simulink model "Van0"  (R2024b)
settings: Solver=ode3  StartTime=0.0  StopTime=10  FixedStep=0.001  RelTol=1e-3
Description:
  | 原始版本
settings Model: PacingRate=1000  Creator=繁星  LastModifiedBy=14422
settings SolverCC: ShapePreserveControl=EnableAll  ZeroCrossAlgorithm=Adaptive
settings DataIOCC: ReturnWorkspaceOutputs=off
settings OptimizationCC: ReuseModelBlockBuffer=off
settings ModelReferenceCC: EnableRefExpFcnMdlSchedulingChecks=on
settings RTWCC: GPUComputeCapability=3.5

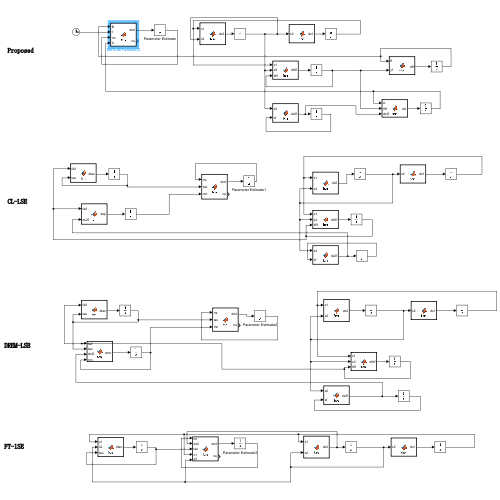
[thumbnail: Simulink's stored preview of the top-level diagram]
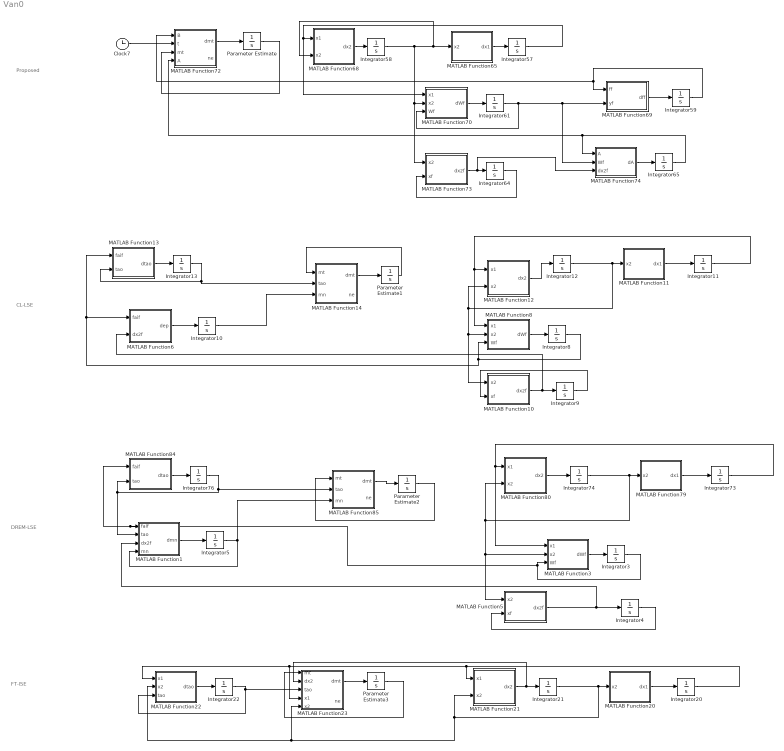
== system Van0 ==
  note: Proposed
  note: CL-LSE
  note: DREM-LSE
  note: FT-lSE
  Clock7 : Clock
  Integrator10 : Integrator  InitialCondition=[0;0;0]
  Integrator{11,20,57,73} (4 alike) : Integrator  InitialCondition=1
  Integrator{3..4,8..9,12,21,58,61,64..65,74} (11 alike) : Integrator
  Integrator13 : Integrator  InitialCondition=1000*eye(3)
  Integrator22 : Integrator  InitialCondition=1000*eye(3)
  Integrator5 : Integrator  InitialCondition=[0;0;0]
  Integrator59 : Integrator  InitialCondition=[1 0 0;0 1 0;0 0 1]*1e-7
  Integrator76 : Integrator  InitialCondition=1000*eye(3)
  MATLAB Function1 : MATLAB Function  TreatAsAtomicUnit=on
  MATLAB Function10 : MATLAB Function  TreatAsAtomicUnit=on
  MATLAB Function11 : MATLAB Function  TreatAsAtomicUnit=on
  MATLAB Function12 : MATLAB Function  TreatAsAtomicUnit=on
  MATLAB Function13 : MATLAB Function  TreatAsAtomicUnit=on
  MATLAB Function14 : MATLAB Function  TreatAsAtomicUnit=on
  MATLAB Function20 : MATLAB Function  TreatAsAtomicUnit=on
  MATLAB Function21 : MATLAB Function  TreatAsAtomicUnit=on
  MATLAB Function22 : MATLAB Function  TreatAsAtomicUnit=on
  MATLAB Function23 : MATLAB Function  TreatAsAtomicUnit=on
  MATLAB Function3 : MATLAB Function  TreatAsAtomicUnit=on
  MATLAB Function5 : MATLAB Function  TreatAsAtomicUnit=on
  MATLAB Function6 : MATLAB Function  TreatAsAtomicUnit=on
  MATLAB Function65 : MATLAB Function  TreatAsAtomicUnit=on
  MATLAB Function68 : MATLAB Function  TreatAsAtomicUnit=on
  MATLAB Function69 : MATLAB Function  TreatAsAtomicUnit=on
  MATLAB Function70 : MATLAB Function  TreatAsAtomicUnit=on
  MATLAB Function72 : MATLAB Function  TreatAsAtomicUnit=on
  MATLAB Function73 : MATLAB Function  TreatAsAtomicUnit=on
  MATLAB Function74 : MATLAB Function  TreatAsAtomicUnit=on
  MATLAB Function79 : MATLAB Function  TreatAsAtomicUnit=on
  MATLAB Function8 : MATLAB Function  TreatAsAtomicUnit=on
  MATLAB Function80 : MATLAB Function  TreatAsAtomicUnit=on
  MATLAB Function84 : MATLAB Function  TreatAsAtomicUnit=on
  MATLAB Function85 : MATLAB Function  TreatAsAtomicUnit=on
  Parameter Estimate : Integrator
  Parameter Estimate1 : Integrator  InitialCondition=[0.5;-1;1]*0
  Parameter Estimate2 : Integrator  InitialCondition=[0.5;-1;1]*0
  Parameter Estimate3 : Integrator  InitialCondition=[0.5;-1;1]*0
  wires:
  MATLAB Function73/1(dx2f) -> MATLAB Function74/3(dx2f), Integrator64/1
  MATLAB Function80/1(dx2) -> Integrator74/1
  MATLAB Function79/1(dx1) -> Integrator73/1
  MATLAB Function84/1(dtao) -> Integrator76/1
  Parameter Estimate2/1 -> MATLAB Function85/1(mt)
  Parameter Estimate/1 -> MATLAB Function72/3(mt)
  Integrator76/1 -> MATLAB Function1/2(tao), MATLAB Function84/2(tao), MATLAB Function85/2(tao)
  MATLAB Function85/1(dmt) -> Parameter Estimate2/1
  MATLAB Function69/1(dff) -> Integrator59/1
  Integrator59/1 -> MATLAB Function72/1(B), MATLAB Function69/1(ff)
  MATLAB Function68/1(dx2) -> Integrator58/1
  MATLAB Function70/1(dWf) -> Integrator61/1
  Integrator61/1 -> MATLAB Function70/3(Wf), MATLAB Function74/2(Wf), MATLAB Function69/2(yf)
  MATLAB Function74/1(dA) -> Integrator65/1
  Integrator65/1 -> MATLAB Function72/4(A), MATLAB Function74/1(A)
  MATLAB Function65/1(dx1) -> Integrator57/1
  Integrator64/1 -> MATLAB Function73/2(xf)
  MATLAB Function72/1(dmt) -> Parameter Estimate/1
  Clock7/1 -> MATLAB Function72/2(t)
  Integrator58/1 -> MATLAB Function68/2(x2), MATLAB Function65/1(x2), MATLAB Function70/2(x2), MATLAB Function73/1(x2)
  MATLAB Function3/1(dWf) -> Integrator3/1
  Integrator4/1 -> MATLAB Function5/2(xf)
  MATLAB Function5/1(dx2f) -> MATLAB Function1/3(dx2f), Integrator4/1
  Integrator3/1 -> MATLAB Function84/1(faif), MATLAB Function1/1(faif), MATLAB Function3/3(Wf)
  MATLAB Function1/1(dmn) -> Integrator5/1
  Integrator5/1 -> MATLAB Function1/4(mn), MATLAB Function85/3(mn)
  Integrator74/1 -> MATLAB Function5/1(x2), MATLAB Function3/2(x2), MATLAB Function80/2(x2), MATLAB Function79/1(x2)
  Integrator9/1 -> MATLAB Function10/2(xf)
  MATLAB Function8/1(dWf) -> Integrator8/1
  MATLAB Function6/1(dep) -> Integrator10/1
  MATLAB Function10/1(dx2f) -> Integrator9/1, MATLAB Function6/2(dx2f)
  Parameter Estimate1/1 -> MATLAB Function14/1(mt)
  MATLAB Function11/1(dx1) -> Integrator11/1
  MATLAB Function14/1(dmt) -> Parameter Estimate1/1
  Integrator12/1 -> MATLAB Function10/1(x2), MATLAB Function8/2(x2), MATLAB Function12/2(x2), MATLAB Function11/1(x2)
  MATLAB Function13/1(dtao) -> Integrator13/1
  Integrator8/1 -> MATLAB Function8/3(Wf), MATLAB Function13/1(faif), MATLAB Function6/1(faif)
  MATLAB Function12/1(dx2) -> Integrator12/1
  Integrator10/1 -> MATLAB Function14/3(mn)
  Integrator22/1 -> MATLAB Function22/3(tao), MATLAB Function23/3(tao)
  Parameter Estimate3/1 -> MATLAB Function23/1(mt)
  MATLAB Function20/1(dx1) -> Integrator20/1
  MATLAB Function23/1(dmt) -> Parameter Estimate3/1
  Integrator21/1 -> MATLAB Function20/1(x2), MATLAB Function23/5(x2), MATLAB Function22/2(x2), MATLAB Function21/2(x2)
  MATLAB Function22/1(dtao) -> Integrator22/1
  MATLAB Function21/1(dx2) -> MATLAB Function23/2(dx2), Integrator21/1
  Integrator13/1 -> MATLAB Function14/2(tao), MATLAB Function13/2(tao)
  Integrator57/1 -> MATLAB Function70/1(x1), MATLAB Function68/1(x1)
  Integrator11/1 -> MATLAB Function8/1(x1), MATLAB Function12/1(x1)
  Integrator73/1 -> MATLAB Function3/1(x1), MATLAB Function80/1(x1)
  Integrator20/1 -> MATLAB Function22/1(x1), MATLAB Function23/4(x1), MATLAB Function21/1(x1)

== matlab function Van0/MATLAB Function8 ==
  data: x1 input; dWf output; x2 input; Wf input
function dWf  = fcn(x1,x2,Wf)

A=[-x1,x2,-x1*x1*x2];
dWf=-0.1*Wf+A;

== matlab function Van0/MATLAB Function20 ==
  data: x2 input; dx1 output
function dx1 = fcn(x2)
dx1=x2;

== matlab function Van0/MATLAB Function21 ==
  data: x1 input; x2 input; dx2 output
function dx2  = fcn(x1,x2)


% dx2=[-x1,x2,-x1*x1*x2]*e-x1-x2;
theta=[0.5;-1;1];
% dx2=[-x1,x2,-x1*x1*x2]*theta;

x=[x1;x2];
% u=ddxr(2)-[4 4]*(x-xr)-[-x1,x2,-x1*x1*x2]*mtheta;
%dx2=-[-x1,x2,-x1*x1*x2]*e+ddxr(2)-[4 4]*(x-xr);
dx2=[-x1,x2,-x1*x1*x2]*theta;
% theta=[0.5;-1];
% dx2=[-x1,x2]*theta;

== matlab function Van0/MATLAB Function22 ==
  data: x1 input; x2 input; dtao output; tao input
function dtao = fcn(x1,x2,tao)


fai=[-x1,x2,-x1*x1*x2];

dtao=-tao*fai'*fai*tao;

== matlab function Van0/MATLAB Function23 ==
  data: dmt output size=3,1; mt input; dx2 input; ne output; tao input; x1 input; x2 input
function [dmt,ne]   = fcn(mt,dx2,tao,x1,x2)



theta=[0.5;-1;1];
fai=[-x1,x2,-x1*x1*x2];


  ne=norm(theta-mt);


dmt=tao*fai'*(dx2-fai*mt);

== matlab function Van0/MATLAB Function65 ==
  data: x2 input; dx1 output
function dx1 = fcn(x2)
dx1=x2;

== matlab function Van0/MATLAB Function68 ==
  data: x1 input; x2 input size=1; dx2 output size=1
function dx2  = fcn(x1,x2)


theta=[0.5;-1;1];

u=0;

dx2=[-x1,x2,-x1*x1*x2]*theta+u;

== matlab function Van0/MATLAB Function69 ==
  data: ff input; dff output; yf input
function dff = fcn(ff,yf)


dff=-1*ff+yf'*yf;

== matlab function Van0/MATLAB Function70 ==
  data: x1 input; dWf output; x2 input; Wf input
function dWf  = fcn(x1,x2,Wf)

A=[-x1,x2,-x1*x1*x2];
dWf=-0.1*Wf+A;

== matlab function Van0/MATLAB Function72 ==
  data: B input; dmt output size=3,1; t input; mt input; A input size=3,1; ne output
function [dmt,ne]    = fcn(B,t,mt,A)





theta=[0.5;-1;1];
k1=1e-7;
ne=norm(theta-mt);%Parameter estimation error norm

k=0.2;
Tp=2;%Predefined constant

ee=B\A-(1*eye(3)-k1*eye(3)*exp(-1*t)/B)*mt;

%Parameter update law
dmt=exp(abs(ee).^k).*sign(ee).*abs(ee).^(1-k)/(k*Tp);

== matlab function Van0/MATLAB Function73 ==
  data: x2 input; xf input; dx2f output
function dx2f  = fcn(x2,xf)


dx2f=-0.1*xf+x2;

== matlab function Van0/MATLAB Function74 ==
  data: A input; dA output; Wf input; dx2f input
function dA  = fcn(A,Wf,dx2f)


dA=-1*A+Wf'*(dx2f);

== matlab function Van0/MATLAB Function79 ==
  data: x2 input; dx1 output
function dx1 = fcn(x2)
dx1=x2;

== matlab function Van0/MATLAB Function80 ==
  data: x1 input; x2 input; dx2 output
function dx2  = fcn(x1,x2)


% dx2=[-x1,x2,-x1*x1*x2]*e-x1-x2;
theta=[0.5;-1;1];
% dx2=[-x1,x2,-x1*x1*x2]*theta;

x=[x1;x2];
% u=ddxr(2)-[4 4]*(x-xr)-[-x1,x2,-x1*x1*x2]*mtheta;
%dx2=-[-x1,x2,-x1*x1*x2]*e+ddxr(2)-[4 4]*(x-xr);
dx2=[-x1,x2,-x1*x1*x2]*theta;
% theta=[0.5;-1];
% dx2=[-x1,x2]*theta;

== matlab function Van0/MATLAB Function84 ==
  data: faif input; dtao output; tao input
function dtao = fcn(faif,tao)


dtao=-tao*faif'*faif*tao;

== matlab function Van0/MATLAB Function85 ==
  data: dmt output size=3,1; mt input; tao input; mn input; ne output
function [dmt,ne]   = fcn(mt,tao,mn)



theta=[0.5;-1;1];

gama=100;

  ne=norm(theta-mt);







A=eye(3)-inv(1000*eye(3))*tao;
adj_A = zeros(3,3);

% 计算每个余因子元素（展开循环优化性能）
adj_A(1,1) =  det(A([2,3], [2,3])) * (-1)^(1+1);
adj_A(1,2) = det(A([2,3], [1,3])) * (-1)^(1+2);
adj_A(1,3) =  det(A([2,3], [1,2])) * (-1)^(1+3);

adj_A(2,1) = det(A([1,3], [2,3])) * (-1)^(2+1);
adj_A(2,2) =  det(A([1,3], [1,3])) * (-1)^(2+2);
adj_A(2,3) = det(A([1,3], [1,2])) * (-1)^(2+3);

adj_A(3,1) =  det(A([1,2], [2,3])) * (-1)^(3+1);
adj_A(3,2) = det(A([1,2], [1,3])) * (-1)^(3+2);
adj_A(3,3) =  det(A([1,2], [1,2])) * (-1)^(3+3);

% 转置余因子矩阵得到伴随矩阵
adjoint1 = adj_A';



fai=adjoint1*mn;
deta=det(eye(3)-inv(1000*eye(3))*tao);
dmt=gama*deta*(fai-deta*mt);

== matlab function Van0/MATLAB Function1 ==
  data: faif input; dmn output; tao input; dx2f input; mn input
function dmn = fcn(faif,tao,dx2f,mn)



dmn=tao*faif'*(dx2f-faif*mn);

== matlab function Van0/MATLAB Function3 ==
  data: x1 input; dWf output; x2 input; Wf input
function dWf  = fcn(x1,x2,Wf)

A=[-x1,x2,-x1*x1*x2];
dWf=-0.1*Wf+A;

== matlab function Van0/MATLAB Function5 ==
  data: x2 input; xf input; dx2f output
function dx2f  = fcn(x2,xf)


dx2f=-0.1*xf+x2;

== matlab function Van0/MATLAB Function10 ==
  data: x2 input; xf input; dx2f output
function dx2f  = fcn(x2,xf)


dx2f=-0.1*xf+x2;

== matlab function Van0/MATLAB Function11 ==
  data: x2 input; dx1 output
function dx1 = fcn(x2)
dx1=x2;

== matlab function Van0/MATLAB Function12 ==
  data: x1 input; x2 input; dx2 output
function dx2  = fcn(x1,x2)


% dx2=[-x1,x2,-x1*x1*x2]*e-x1-x2;
theta=[0.5;-1;1];
% dx2=[-x1,x2,-x1*x1*x2]*theta;

x=[x1;x2];
% u=ddxr(2)-[4 4]*(x-xr)-[-x1,x2,-x1*x1*x2]*mtheta;
%dx2=-[-x1,x2,-x1*x1*x2]*e+ddxr(2)-[4 4]*(x-xr);
dx2=[-x1,x2,-x1*x1*x2]*theta;
% theta=[0.5;-1];
% dx2=[-x1,x2]*theta;

== matlab function Van0/MATLAB Function13 ==
  data: faif input; dtao output; tao input
function dtao = fcn(faif,tao)


dtao=-tao*faif'*faif*tao;

== matlab function Van0/MATLAB Function14 ==
  data: dmt output size=3,1; mt input; tao input; mn input; ne output
function [dmt,ne]   = fcn(mt,tao,mn)



theta=[0.5;-1;1];

Q=inv(tao)-inv(1000*eye(3));

gama=100;

ne=norm(theta-mt);
dmt=gama*tao*(mn-Q*mt);

== matlab function Van0/MATLAB Function6 ==
  data: faif input; dep output; dx2f input
function dep = fcn(faif,dx2f)



dep=faif'*dx2f;
